simulink model "innerLoop_currentControl"  (R2023b)
settings: Solver=ode1  StartTime=0.0  StopTime=Tsim_inLoop  FixedStep=Tstep  RelTol=1e-3
values from neighbouring files (symbols this model uses):
  ILnom = 5    [DCDC_param.m]
  L = 1.1*max(VinNom*D*Tsw / dIL, VinNom*(1-D)*Tsw / dIL)    [DCDC_param.m]    (also in inductance.m = 0.002)
  RserL = L * (0.14/5e-3)    [DCDC_param.m]
  VinNom = 30    [DCDC_param.m]
  VoutNom = 50    [DCDC_param.m]
undefined symbols (not defined in the file or in its folder): den_aaf, kaw_i, ki_i, kp_i, kpf_i, num_aaf, Tsim_inLoop, VLlim
libraries: simulink x1
settings Model: Creator=nicholas  LastModifiedBy=nicholas

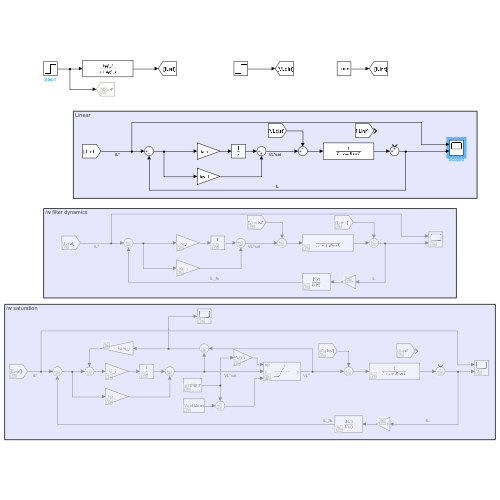
[thumbnail: Simulink's stored preview of the top-level diagram]
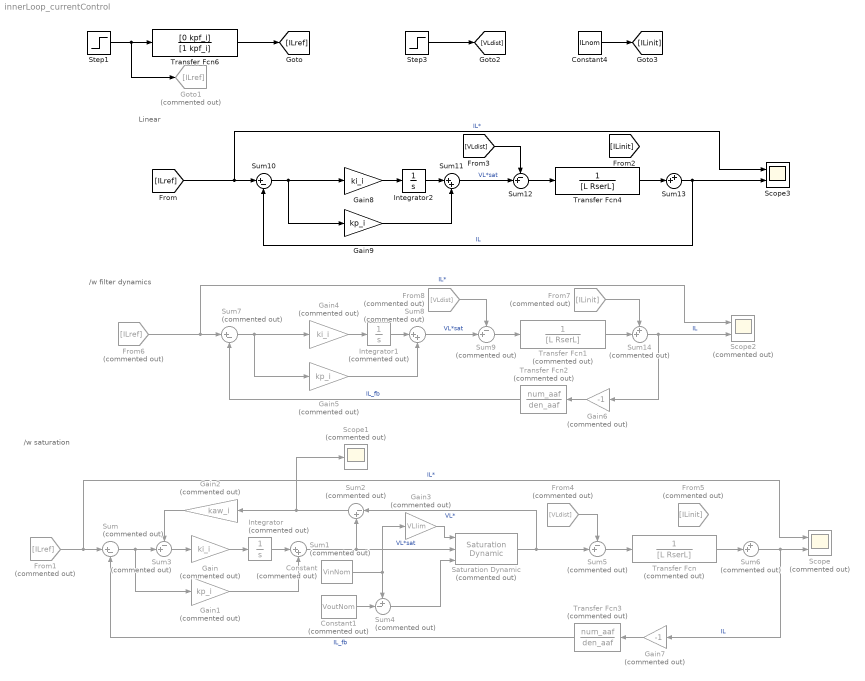
== system innerLoop_currentControl ==
  note: /w saturation
  note: /w filter dynamics
  note: Linear
  Constant : Constant  Commented=on  Value=VinNom
  Constant1 : Constant  Commented=on  Value=VoutNom
  Constant4 : Constant  Value=ILnom
  From1 : From  Commented=on  GotoTag=ILref
  From4 : From  Commented=on  GotoTag=VLdist
  From5 : From  Commented=on  GotoTag=ILinit
  From6 : From  Commented=on  GotoTag=ILref
  From7 : From  Commented=on  GotoTag=ILinit
  From8 : From  Commented=on  GotoTag=VLdist
  Gain : Gain  Commented=on  Gain=ki_i
  Gain1 : Gain  Commented=on  Gain=kp_i
  Gain2 : Gain  Commented=on  Gain=kaw_i
  Gain3 : Gain  Commented=on  Gain=VLlim
  Gain4 : Gain  Commented=on  Gain=ki_i
  Gain5 : Gain  Commented=on  Gain=kp_i
  Gain6 : Gain  Commented=on  Gain=-1
  Gain7 : Gain  Commented=on  Gain=-1
  Gain8 : Gain  Gain=ki_i
  Gain9 : Gain  Gain=kp_i
  Goto1 : Goto  Commented=on  GotoTag=ILref
  Integrator : Integrator  Commented=on
  Integrator1 : Integrator  Commented=on
  Integrator2 : Integrator
  Saturation Dynamic : simulink/Discontinuities/Saturation Dynamic  Commented=on  OutMin=[]  OutMax=[]  OutDataTypeStr=Inherit: Same as second input  OutDataType=fixdt(1, 16)  OutScaling=2^-10  DoSatur=off
  Scope : Scope  Commented=on  NumInputPorts=2
  Scope1 : Scope  Commented=on
  Scope2 : Scope  Commented=on  NumInputPorts=2
  Scope3 : Scope  NumInputPorts=2
  Step1 : Step  Time=0.02  After=ILnom  SampleTime=0
  Step3 : Step  Time=Tsim_inLoop/2  After=VinNom/4  SampleTime=0
  Sum : Sum  Commented=on  Inputs=|+-
  Sum1 : Sum  Commented=on  Inputs=|++
  Sum10 : Sum  Inputs=|+-
  Sum11 : Sum  Inputs=|++
  Sum12 : Sum  Inputs=-+|
  Sum13 : Sum  Inputs=++|
  Sum14 : Sum  Commented=on  Inputs=++|
  Sum2 : Sum  Commented=on  Inputs=|-+
  Sum3 : Sum  Commented=on  Inputs=-+|
  Sum4 : Sum  Commented=on  Inputs=+-|
  Sum5 : Sum  Commented=on  Inputs=-+|
  Sum6 : Sum  Commented=on  Inputs=++|
  Sum7 : Sum  Commented=on  Inputs=|+-
  Sum8 : Sum  Commented=on  Inputs=|++
  Sum9 : Sum  Commented=on  Inputs=-+|
  Transfer Fcn : TransferFcn  Commented=on  Denominator=[L RserL]
  Transfer Fcn1 : TransferFcn  Commented=on  Denominator=[L RserL]
  Transfer Fcn2 : TransferFcn  Commented=on  Numerator=num_aaf  Denominator=den_aaf
  Transfer Fcn3 : TransferFcn  Commented=on  Numerator=num_aaf  Denominator=den_aaf
  Transfer Fcn4 : TransferFcn  Denominator=[L RserL]
  Transfer Fcn6 : TransferFcn  Numerator=[0 kpf_i]  Denominator=[1 kpf_i]
  wires:
  Sum/1 -> Sum3/2, Gain1/1
  Gain/1 -> Integrator/1
  Integrator/1 -> Sum1/1
  Gain1/1 -> Sum1/2
  Sum1/1 -> Saturation Dynamic/2, Sum2/2  "VL*sat"
  Saturation Dynamic/1 -> Sum5/2, Sum2/1  "VL*"
  Sum3/1 -> Gain/1
  Gain2/1 -> Sum3/1
  Sum4/1 -> Saturation Dynamic/3
  Constant/1 -> Gain3/1, Sum4/1
  Constant1/1 -> Sum4/2
  Gain3/1 -> Saturation Dynamic/1
  Sum2/1 -> Scope1/1, Gain2/1
  From1/1 -> Scope/1, Sum/1  "IL*"
  [ILref] -> Scope3/1, Sum10/1  "IL*"
  Sum10/1 -> Gain8/1, Gain9/1
  Integrator2/1 -> Sum11/1
  Gain8/1 -> Integrator2/1
  Gain9/1 -> Sum11/2
  Sum11/1 -> Sum12/2  "VL*sat"
  Transfer Fcn4/1 -> Sum13/2
  Sum12/1 -> Transfer Fcn4/1
  Sum13/1 -> Sum10/2, Scope3/2  "IL"
  Transfer Fcn6/1 -> [ILref]
  [VLdist] -> Sum12/1
  From4/1 -> Sum5/1
  Sum5/1 -> Transfer Fcn/1
  Transfer Fcn/1 -> Sum6/2
  Sum6/1 -> Scope/2, Gain7/1  "IL"
  Constant4/1 -> [ILinit]
  Step3/1 -> [VLdist]
  Transfer Fcn1/1 -> Sum14/2
  Gain5/1 -> Sum8/2
  Integrator1/1 -> Sum8/1
  Sum9/1 -> Transfer Fcn1/1
  Sum8/1 -> Sum9/2  "VL*sat"
  Sum7/1 -> Gain4/1, Gain5/1
  From8/1 -> Sum9/1
  Gain4/1 -> Integrator1/1
  From6/1 -> Scope2/1, Sum7/1  "IL*"
  Sum14/1 -> Gain6/1, Scope2/2  "IL"
  From7/1 -> Sum14/1
  Transfer Fcn2/1 -> Sum7/2  "IL_fb"
  Gain6/1 -> Transfer Fcn2/1
  Gain7/1 -> Transfer Fcn3/1
  Transfer Fcn3/1 -> Sum/2  "IL_fb"
  Step1/1 -> Transfer Fcn6/1, Goto1/1
